simulink model "example01b"  (R2022a)
settings: Solver=VariableStepAuto  StartTime=0.0  StopTime=10.0  RelTol=1e-3
settings Model: Creator=cunis  LastModifiedBy=cunis

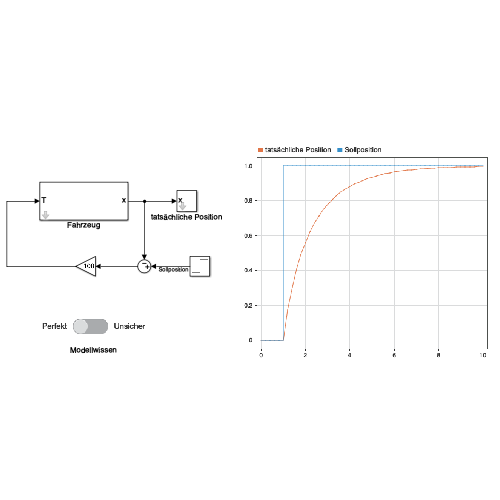
[thumbnail: Simulink's stored preview of the top-level diagram]
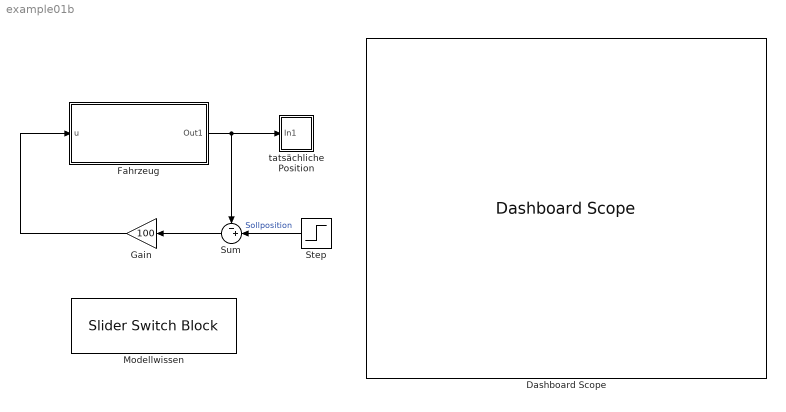
== system example01b ==
  Dashboard Scope : DashboardScope
  Fahrzeug : Subsystem
      mask Display:
      | port_label('input', 1, 'T');
      | port_label('output', 1, 'x');
  Gain : Gain  Gain=100
  Modellwissen : SliderSwitchBlock  LabelPosition=Hide
      settings: Values={{'Perfekt', 'Unsicher'}, [0 1]}
  Step : Step  SampleTime=0
  Sum : Sum  Inputs=-+|
  tatsächliche Position : Subsystem
      mask Display: port_label('input', 1, 'x');
  wires:
  Fahrzeug/1(Out1) -> tatsächliche Position/1(In1), Sum/1
  Step/1 -> Sum/2  "Sollposition"
  Sum/1 -> Gain/1
  Gain/1 -> Fahrzeug/1(u)

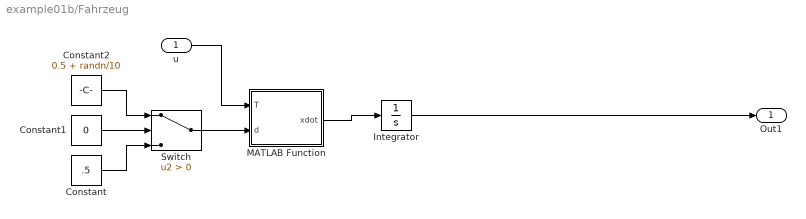
== system example01b/Fahrzeug ==
  u : Inport
  Constant : Constant  Value=.5
  Constant1 : Constant  Value=0
  Constant2 : Constant  Value=0.5 + randn/10
  Integrator : Integrator
  MATLAB Function : MATLAB Function  TreatAsAtomicUnit=on
  Switch : Switch  Criteria=u2 > Threshold  SaturateOnIntegerOverflow=off  InputSameDT=off
  Out1 : Outport
  wires:
  u/1 -> MATLAB Function/1(T)
  MATLAB Function/1(xdot) -> Integrator/1
  Integrator/1 -> Out1/1
  Switch/1 -> MATLAB Function/2(d)
  Constant2/1 -> Switch/1
  Constant/1 -> Switch/3
  Constant1/1 -> Switch/2

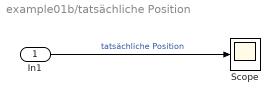
== system example01b/tatsächliche Position ==
  In1 : Inport
  Scope : Scope
  wires:
  In1/1 -> Scope/1  "tatsächliche Position"

== matlab function example01b/Fahrzeug/MATLAB Function ==
  data: T input; xdot output; d input
function xdot = fcn(T, d)

xdot = sign(T)*(exp(abs(T)/100-d) - exp(-d))/(exp(d) - exp(-d));

end
